simulink model "chapter4_P2"  (R2017a)
settings: Solver=ode1  StartTime=0.0  StopTime=inf  FixedStep=0.001  RelTol=1e-3  EnableMultiTasking=on
undefined symbols (not defined in the file or in its folder): k13, k23
libraries: c6xlib x2
Description:
  | Real-Time Van der Pol Simulation
  | 
  | This demonstration shows a real-time version of the Simulink(R) Van der Pol
  | simulation demo. This model does not need any external signals, so it does
  | not need any data acquisition hardware or driver. This makes the model ideal
  | for first experiments with Real-Time Windows Target(TM), without need to
  | worry about proper I/O hardware configuration.
  | 
  | How to run this demo:
  | 
  |   1. Build the model using Tools -> Real-Time Workshop -> Build Model.
  |   2. Connect to the real-time code using Simulation -> Connect to target.
  |   3. Start the real-time execution using Simulation -> Start real-time code.
settings Model: SimulationMode=external  ExtModeTrigDuration=50000  Creator=Houska  LastModifiedBy=lwang114
settings DataIOCC: SaveFormat=Array  SignalLoggingSaveFormat=ModelDataLogs  SignalLoggingName=logsOut
settings OptimizationCC: ExpressionDepthLimit=2147483647  InitFltsAndDblsToZero=on  EfficientMapNaN2IntZero=off
settings DebuggingCC: UnderspecifiedInitializationDetection=Classic  MergeDetectMultiDrivingBlocksExec=none  SignalResolutionControl=TryResolveAllWithWarning  FcnCallInpInsideContextMsg=warning  StateNameClashWarn=warning  SFUnexpectedBacktrackingDiag=warning  SFNoUnconditionalDefaultTransitionDiag=warning  SFExecutionAtInitializationDiag=none
settings ModelReferenceCC: PropagateSignalLabelsOutOfModel=off
settings RTWCC: SystemTargetFile=sldrt.tlc  TemplateMakefile=sldrt.tmf  Description=Simulink Desktop Real-Time  RTWCompilerOptimization=on
settings CodeAppCC: MaxIdLength=95
settings SimulinkDesktopRealTimeCC: TargetPreCompLibLocation=C:\MATLABR2017a\toolbox\sldrt\lib\win64  TargetLangStandard=C89/C90 (ANSI)  SupportVariableSizeSignals=off
settings ConfigComp: CovMetricSettings=dw  CovHtmlReporting=on  CovSaveCumulativeToWorkspaceVar=on  CovSaveSingleToWorkspaceVar=on  CovExternalEMLEnable=off  CovSFcnEnable=off

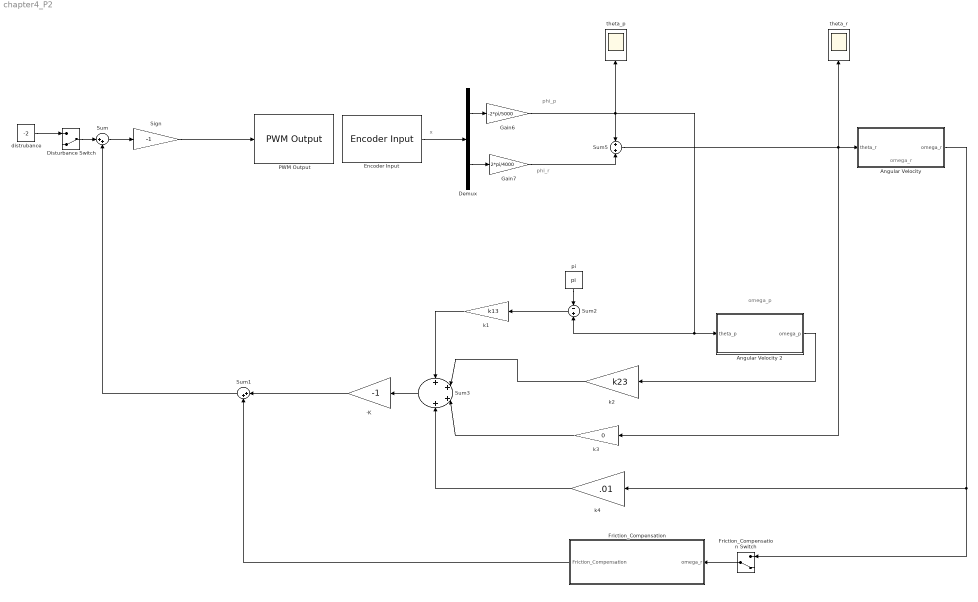
== system chapter4_P2 ==
  note: x
  note: phi_p
  note: phi_r
  note: omega_p
  note: omega_r
  -K : Gain  Gain=-1
  Angular Velocity : Subsystem
  Angular Velocity 2 : Subsystem
  Demux : Demux  Outputs=2
  Disturbance Switch : ManualSwitch  CurrentSetting=0
  Encoder Input : c6xlib/Encoder Input  baseAddr=0x378  channels=[0 1]  sampleTime=str2num(get_param(bdroot, 'FixedStep'))
  Friction_Compensation : Subsystem
  Friction_Compensation Switch : ManualSwitch  CurrentSetting=0
  Gain6 : Gain  Gain=-2*pi/5000
  Gain7 : Gain  Gain=2*pi/4000
  PWM Output : c6xlib/PWM Output  baseAddr=0x378  channels=0  initialOutputs=0  finalOutputs=0  sampleTime=str2num(get_param(bdroot, 'FixedStep'))
  Sign : Gain  Gain=-1
  Sum : Sum  Inputs=|++
  Sum1 : Sum  Inputs=|++
  Sum2 : Sum  Inputs=-+
  Sum3 : Sum  Inputs=++++
  Sum5 : Sum
  distrubance : Constant  Value=-2
  "k1 " : Gain  Gain=k13
  "k2 " : Gain  Gain=k23
  k3 : Gain  Gain=0
  k4 : Gain  Gain=.01
  pi : Constant  Value=pi
  theta_p : Scope
  theta_r : Scope
  wires:
  Demux/1 -> Gain6/1
  Gain7/1 -> Sum5/2
  Demux/2 -> Gain7/1
  Encoder Input/1 -> Demux/1
  Disturbance Switch/1 -> Sum/1
  distrubance/1 -> Disturbance Switch/1
  -K/1 -> Sum1/1
  Friction_Compensation/1(Friction_Compensation) -> Sum1/2
  Friction_Compensation Switch/1 -> Friction_Compensation/1(omega_r)
  Sign/1 -> PWM Output/1
  Sum/1 -> Sign/1
  k4/1 -> Sum3/4
  k3/1 -> Sum3/3
  Sum5/1 -> theta_r/1, Angular Velocity/1(theta_r), k3/1
  Angular Velocity 2/1(omega_p) -> "k2 "/1
  Sum3/1 -> -K/1
  "k2 "/1 -> Sum3/2
  "k1 "/1 -> Sum3/1
  Angular Velocity/1(omega_r) -> Friction_Compensation Switch/1, k4/1
  Sum2/1 -> "k1 "/1
  pi/1 -> Sum2/1
  Gain6/1 -> Sum2/2, Angular Velocity 2/1(theta_p), theta_p/1, Sum5/1
  Sum1/1 -> Sum/2

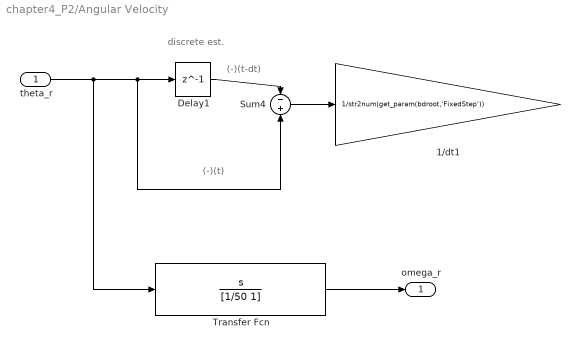
== system chapter4_P2/Angular Velocity ==
  note: (-)(t-dt)
  note: discrete est.
  note: (-)(t)
  theta_r : Inport
  1/dt1 : Gain  Gain=1/str2num(get_param(bdroot,'FixedStep'))
  Delay1 : Delay  DelayLength=1  InitialCondition=0
  Sum4 : Sum  Inputs=-+
  Transfer Fcn : TransferFcn  Numerator=[1 0]  Denominator=[1/50 1]
  omega_r : Outport
  wires:
  theta_r/1 -> Transfer Fcn/1, Delay1/1, Sum4/2
  Sum4/1 -> 1/dt1/1
  Delay1/1 -> Sum4/1
  Transfer Fcn/1 -> omega_r/1

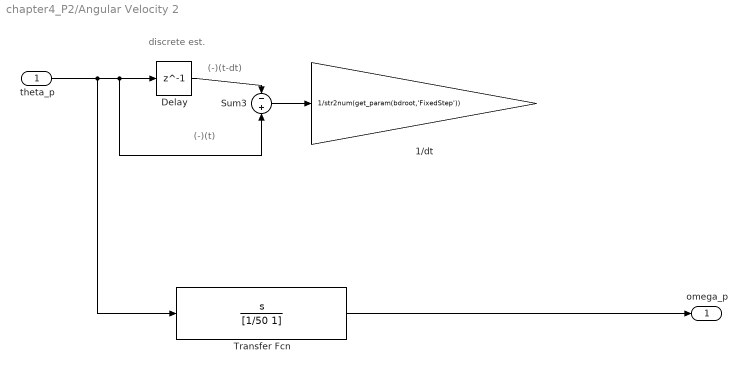
== system chapter4_P2/Angular Velocity 2 ==
  note: (-)(t)
  note: discrete est.
  note: (-)(t-dt)
  theta_p : Inport
  1/dt : Gain  Gain=1/str2num(get_param(bdroot,'FixedStep'))
  Delay : Delay  DelayLength=1  InitialCondition=0
  Sum3 : Sum  Inputs=-+
  Transfer Fcn : TransferFcn  Numerator=[1 0]  Denominator=[1/50 1]
  omega_p : Outport
  wires:
  Delay/1 -> Sum3/1
  Sum3/1 -> 1/dt/1
  theta_p/1 -> Transfer Fcn/1, Delay/1, Sum3/2
  Transfer Fcn/1 -> omega_p/1

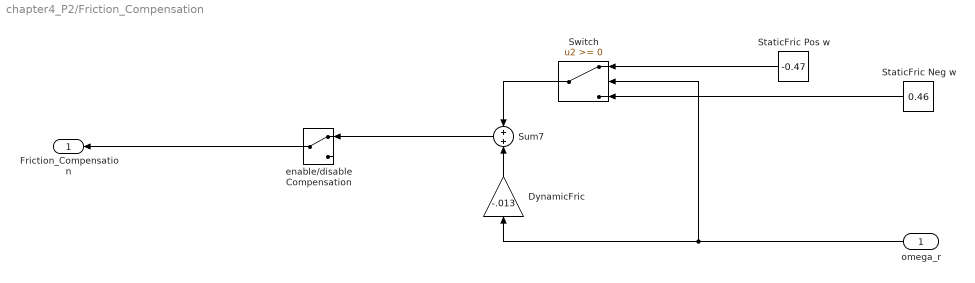
== system chapter4_P2/Friction_Compensation ==
  omega_r : Inport
  DynamicFric : Gain  Gain=-.013
  "StaticFric Neg w " : Constant  Value=0.46
  StaticFric Pos w : Constant  Value=-0.47
  Sum7 : Sum
  Switch : Switch
  enable/disable Compensation : ManualSwitch
  Friction_Compensation : Outport
  wires:
  "StaticFric Neg w "/1 -> Switch/3
  Sum7/1 -> enable/disable Compensation/1
  omega_r/1 -> Switch/2, DynamicFric/1
  enable/disable Compensation/1 -> Friction_Compensation/1
  Switch/1 -> Sum7/1
  StaticFric Pos w/1 -> Switch/1
  DynamicFric/1 -> Sum7/2
